simulink model "BLOC_Electrical_System_supervision"  (R2016a)
settings: Solver=VariableStepAuto  StartTime=0.0  StopTime=10.0  RelTol=1e-3
undefined symbols (not defined in the file): hev_dt, ra_differential_ratio, ra_electrical_machine_speed, ra_transmission_efficiency, syse_electrical_machine_torque_vs_power_speed_nneg, syse_electrical_machine_torque_vs_power_speed_npos, syse_em_in_power, syse_max_charge_current, syse_max_discharge_current, syse_soc_current_limits
settings Model: Creator=Florent  LastModifiedBy=Florent
settings OptimizationCC: DefaultParameterBehavior=Inlined  OptimizeModelRefInitCode=on  LifeSpan=1
settings RTWCC: SystemTargetFile=ert.tlc  TemplateMakefile=ert_default_tmf  GenerateReport=on  IncludeHyperlinkInReport=on  LaunchReport=on  TargetLang=C++  GenerateTraceInfo=on  GenerateTraceReport=on  GenerateTraceReportSl=on  GenerateTraceReportSf=on  GenerateTraceReportEml=on
settings CodeAppCC: ForceParamTrailComments=on  OperatorAnnotations=on  SimulinkDataObjDesc=on  SFDataObjDesc=on  MATLABFcnDesc=on  InsertBlockDesc=on  MATLABSourceComments=on
settings ERTTargetCC: GenerateSampleERTMain=on  MultiInstanceERTCode=on  CodeInterfacePackaging=C++ class  InlinedParameterPlacement=NonHierarchical  RootIOFormat=Structure reference  ERTCustomFileTemplate=example_file_process.tlc

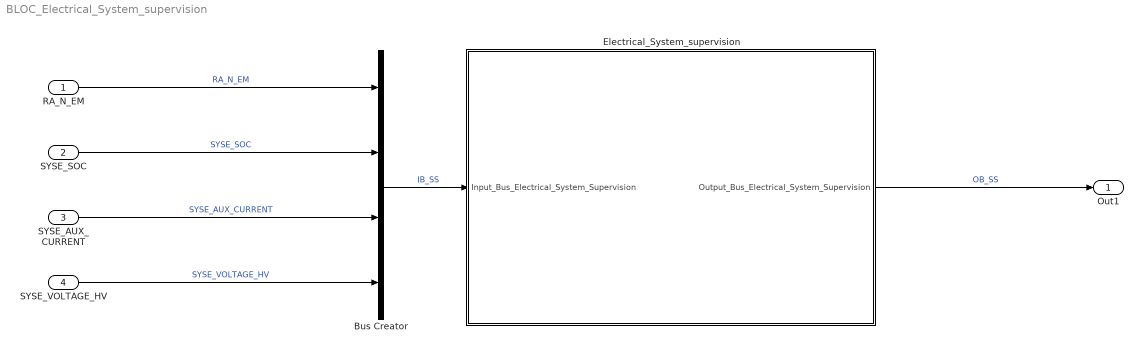
== system BLOC_Electrical_System_supervision ==
  RA_N_EM : Inport
  SYSE_SOC : Inport  Port=2
  SYSE_AUX_CURRENT : Inport  Port=3
  SYSE_VOLTAGE_HV : Inport  Port=4
  Bus Creator : BusCreator  Inputs=4
  Electrical_System_supervision : Subsystem  TreatAsAtomicUnit=on  SystemSampleTime=hev_dt
  Out1 : Outport  PortDimensions=2
  wires:
  Electrical_System_supervision/1(Output_Bus_Electrical_System_Supervision) -> Out1/1  "OB_SS"
  RA_N_EM/1 -> Bus Creator/1  "RA_N_EM"
  SYSE_SOC/1 -> Bus Creator/2  "SYSE_SOC"
  SYSE_VOLTAGE_HV/1 -> Bus Creator/4  "SYSE_VOLTAGE_HV"
  Bus Creator/1 -> Electrical_System_supervision/1(Input_Bus_Electrical_System_Supervision)  "IB_SS"
  SYSE_AUX_CURRENT/1 -> Bus Creator/3  "SYSE_AUX_CURRENT"

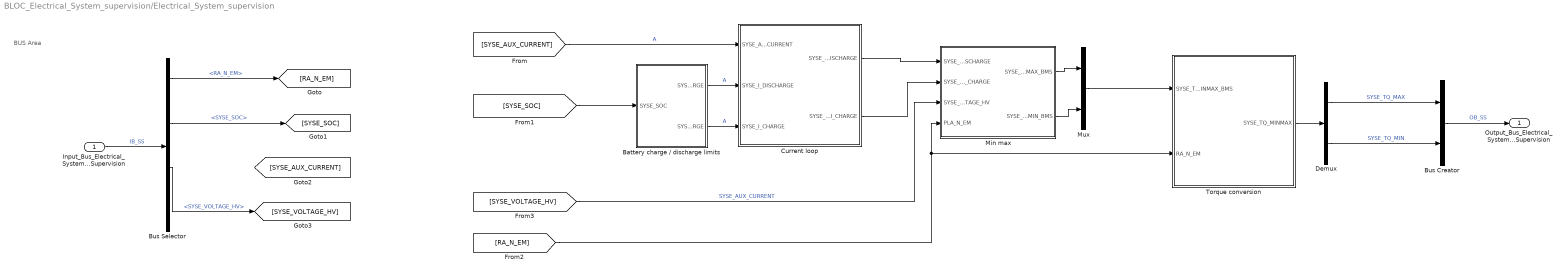
== system BLOC_Electrical_System_supervision/Electrical_System_supervision ==
  note: BUS Area
  Input_Bus_Electrical_System_Supervision : Inport
  Battery charge / discharge limits : Subsystem
  Bus Creator : BusCreator  Inputs=2
  Bus Selector : BusSelector  OutputSignals=RA_N_EM,SYSE_SOC,SYSE_VOLTAGE_HV,SYSE_AUX_CURRENT
  Current loop : Subsystem
  Demux : Demux  Outputs=2
  "Min max " : Subsystem
  Mux : Mux  Inputs=2
  Torque conversion : Subsystem
  Output_Bus_Electrical_System_Supervision : Outport
  wires:
  [SYSE_SOC] -> Battery charge / discharge limits/1(SYSE_SOC)
  Battery charge / discharge limits/1(SYSE_I_DISCHARGE) -> Current loop/2(SYSE_I_DISCHARGE)  "A"
  Battery charge / discharge limits/2(SYSE_I_CHARGE) -> Current loop/3(SYSE_I_CHARGE)  "A"
  Current loop/1(SYSE_EM_I_DISCHARGE) -> "Min max "/1(SYSE_EM_I_DISCHARGE)
  Current loop/2(SYSE_EM_I_CHARGE) -> "Min max "/2(SYSE_EM_I_CHARGE)
  [SYSE_AUX_CURRENT] -> Current loop/1(SYSE_AUX_CURRENT)  "A"
  [SYSE_VOLTAGE_HV] -> "Min max "/3(SYSE_VOLTAGE_HV)  "SYSE_AUX_CURRENT"
  [RA_N_EM] -> "Min max "/4(PLA_N_EM), Torque conversion/2(RA_N_EM)
  "Min max "/2(SYSE_TQ_MIN_BMS) -> Mux/2
  "Min max "/1(SYSE_TQ_MAX_BMS) -> Mux/1
  Mux/1 -> Torque conversion/1(SYSE_TQ_MINMAX_BMS)
  Torque conversion/1(SYSE_TQ_MINMAX) -> Demux/1
  Bus Creator/1 -> Output_Bus_Electrical_System_Supervision/1  "OB_SS"
  Demux/1 -> Bus Creator/1  "SYSE_TQ_MAX"
  Demux/2 -> Bus Creator/2  "SYSE_TQ_MIN"
  Input_Bus_Electrical_System_Supervision/1 -> Bus Selector/1  "IB_SS"
  Bus Selector/1 -> [RA_N_EM]  "<RA_N_EM>"
  Bus Selector/2 -> [SYSE_SOC]  "<SYSE_SOC>"
  ? -> [SYSE_AUX_CURRENT]  "<SYSE_AUX>"
  Bus Selector/3 -> [SYSE_VOLTAGE_HV]  "<SYSE_VOLTAGE_HV>"

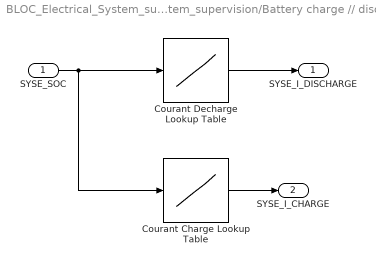
== system BLOC_Electrical_System_supervision/Electrical_System_supervision/Battery charge // discharge limits ==
  SYSE_SOC : Inport
  Courant Charge Lookup Table : Lookup_n-D  NumberOfTableDimensions=1  BreakpointsForDimension1=syse_soc_current_limits/100  Table=-syse_max_charge_current  SampleTime=hev_dt  RndMeth=Simplest  InputSameDT=on
  Courant Decharge Lookup Table : Lookup_n-D  NumberOfTableDimensions=1  BreakpointsForDimension1=syse_soc_current_limits/100  Table=syse_max_discharge_current  SampleTime=hev_dt  RndMeth=Simplest  InputSameDT=on
  SYSE_I_DISCHARGE : Outport
  SYSE_I_CHARGE : Outport  Port=2
  wires:
  SYSE_SOC/1 -> Courant Decharge Lookup Table/1, Courant Charge Lookup Table/1
  Courant Decharge Lookup Table/1 -> SYSE_I_DISCHARGE/1
  Courant Charge Lookup Table/1 -> SYSE_I_CHARGE/1

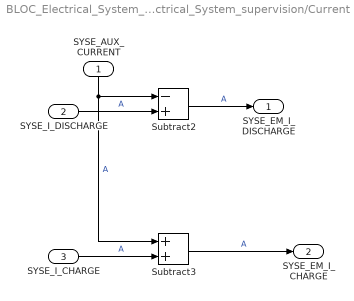
== system BLOC_Electrical_System_supervision/Electrical_System_supervision/Current loop ==
  SYSE_AUX_CURRENT : Inport
  SYSE_I_DISCHARGE : Inport  Port=2
  SYSE_I_CHARGE : Inport  Port=3
  Subtract2 : Sum  Inputs=-+  SampleTime=hev_dt
  Subtract3 : Sum  SampleTime=hev_dt
  SYSE_EM_I_DISCHARGE : Outport
  SYSE_EM_I_CHARGE : Outport  Port=2
  wires:
  SYSE_AUX_CURRENT/1 -> Subtract2/1, Subtract3/1  "A"
  Subtract2/1 -> SYSE_EM_I_DISCHARGE/1  "A"
  SYSE_I_DISCHARGE/1 -> Subtract2/2  "A"
  Subtract3/1 -> SYSE_EM_I_CHARGE/1  "A"
  SYSE_I_CHARGE/1 -> Subtract3/2  "A"

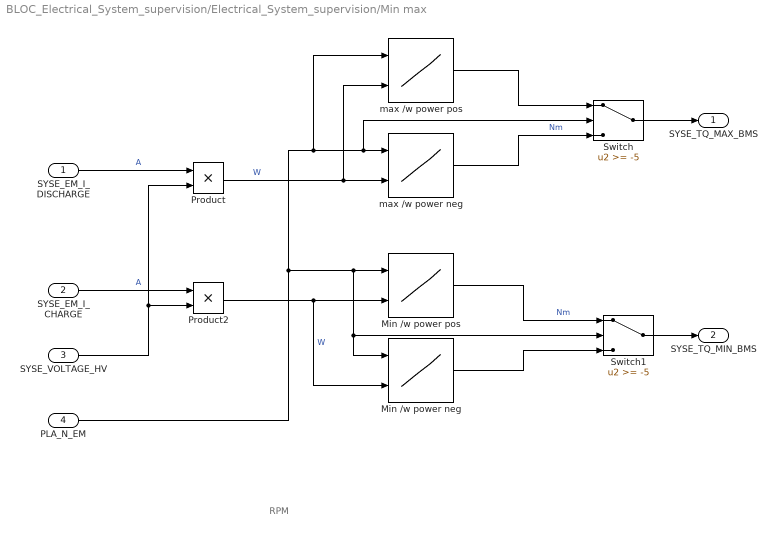
== system BLOC_Electrical_System_supervision/Electrical_System_supervision/Min max  ==
  note: RPM
  SYSE_EM_I_DISCHARGE : Inport
  SYSE_EM_I_CHARGE : Inport  Port=2
  SYSE_VOLTAGE_HV : Inport  Port=3
  PLA_N_EM : Inport  Port=4
  Min /w power neg : Lookup_n-D  BreakpointsForDimension1=ra_electrical_machine_speed(1:10)  BreakpointsForDimension2=syse_em_in_power*1000  Table=syse_electrical_machine_torque_vs_power_speed_nneg  ExtrapMethod=Clip  UseLastTableValue=on  SampleTime=hev_dt  RndMeth=Simplest  InputSameDT=on
  Min /w power pos : Lookup_n-D  BreakpointsForDimension1=ra_electrical_machine_speed(12:20)  BreakpointsForDimension2=syse_em_in_power*1000  Table=syse_electrical_machine_torque_vs_power_speed_npos  ExtrapMethod=Clip  UseLastTableValue=on  SampleTime=hev_dt  RndMeth=Simplest  InputSameDT=on
  Product : Product  SampleTime=hev_dt  RndMeth=Zero
  Product2 : Product  SampleTime=hev_dt  RndMeth=Zero
  Switch : Switch  Threshold=-5  SampleTime=hev_dt
  Switch1 : Switch  Threshold=-5  SampleTime=hev_dt
  max /w power neg : Lookup_n-D  BreakpointsForDimension1=ra_electrical_machine_speed(1:10)  BreakpointsForDimension2=syse_em_in_power*1000  Table=syse_electrical_machine_torque_vs_power_speed_nneg  ExtrapMethod=Clip  UseLastTableValue=on  SampleTime=hev_dt  RndMeth=Simplest  InputSameDT=on
  max /w power pos : Lookup_n-D  BreakpointsForDimension1=ra_electrical_machine_speed(12:20)  BreakpointsForDimension2=syse_em_in_power*1000  Table=syse_electrical_machine_torque_vs_power_speed_npos  ExtrapMethod=Clip  UseLastTableValue=on  SampleTime=hev_dt  RndMeth=Simplest  InputSameDT=on
  SYSE_TQ_MAX_BMS : Outport
  SYSE_TQ_MIN_BMS : Outport  Port=2
  wires:
  PLA_N_EM/1 -> Min /w power pos/1, Min /w power neg/1, Switch1/2, max /w power pos/1, max /w power neg/1, Switch/2
  SYSE_EM_I_DISCHARGE/1 -> Product/1  "A"
  SYSE_EM_I_CHARGE/1 -> Product2/1  "A"
  Product2/1 -> Min /w power pos/2, Min /w power neg/2  "W"
  Product/1 -> max /w power neg/2, max /w power pos/2  "W"
  SYSE_VOLTAGE_HV/1 -> Product2/2, Product/2
  Switch/1 -> SYSE_TQ_MAX_BMS/1
  max /w power pos/1 -> Switch/1
  max /w power neg/1 -> Switch/3  "Nm"
  Min /w power pos/1 -> Switch1/1  "Nm"
  Min /w power neg/1 -> Switch1/3
  Switch1/1 -> SYSE_TQ_MIN_BMS/1

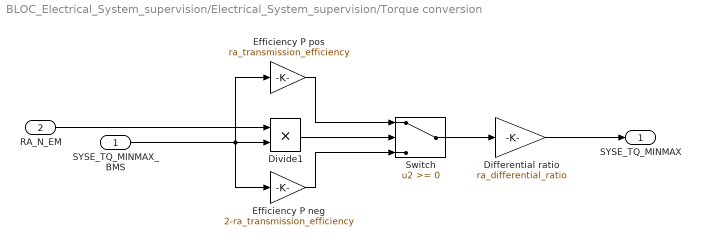
== system BLOC_Electrical_System_supervision/Electrical_System_supervision/Torque conversion ==
  SYSE_TQ_MINMAX_BMS : Inport
  RA_N_EM : Inport  Port=2
  Differential ratio : Gain  Gain=ra_differential_ratio  SampleTime=hev_dt
  Divide1 : Product  SampleTime=hev_dt
  Efficiency P neg : Gain  Gain=2-ra_transmission_efficiency  SampleTime=hev_dt
  Efficiency P pos : Gain  Gain=ra_transmission_efficiency  SampleTime=hev_dt
  Switch : Switch  SampleTime=hev_dt
  SYSE_TQ_MINMAX : Outport
  wires:
  SYSE_TQ_MINMAX_BMS/1 -> Divide1/2, Efficiency P neg/1, Efficiency P pos/1
  Efficiency P pos/1 -> Switch/1
  Efficiency P neg/1 -> Switch/3
  Divide1/1 -> Switch/2
  Switch/1 -> Differential ratio/1
  RA_N_EM/1 -> Divide1/1
  Differential ratio/1 -> SYSE_TQ_MINMAX/1
